simulink model "EiH_VFC_Renew_R2021b"  (R2021b)
settings: Solver=ode4  StartTime=0.0  StopTime=30  FixedStep=0.01  RelTol=1e-3
values from neighbouring files (symbols this model uses):
  denomi_threshold = 1e-8    (= 1e-08)    [param_EiH_VFC.m]
  Keo1 = Keo_Gain    (= 0.5)    [param_EiH_VFC.m]
  Keo2 = Keo_Gain    (= 0.5)    [param_EiH_VFC.m]
  Keo3 = Keo_Gain    (= 0.5)    [param_EiH_VFC.m]
  Keo4 = Keo_Gain    (= 0.5)    [param_EiH_VFC.m]
  Keo5 = Keo_Gain    (= 0.5)    [param_EiH_VFC.m]
  Keo6 = Keo_Gain    (= 0.5)    [param_EiH_VFC.m]
  pco_bar_init = pco_init + [0.15; 0.3; -0.1]    [param_EiH_VFC.m]
  pco_init = [0.0; 0.0; -1.0]    [param_EiH_VFC.m]
  Pinho_Para = [0; 0; 0; lambda_mx; lambda_my]    [param_EiH_VFC.m]
  po = [xo1; yo1; zo1; xo2; yo2; zo2; xo3; yo3; zo3; xo4; yo4; zo4]    [param_EiH_VFC.m]
  pzeta_wo_init = [pwo_init;zetawo_init]    [param_EiH_VFC.m]
  R_threshold = 1e-8    (= 1e-08)    [param_EiH_VFC.m]
  Rco_bar_init = Rfromxi(zetaco_bar_init)    [param_EiH_VFC.m]
  Rco_init = Rfromxi(zetaco_init)    [param_EiH_VFC.m]
  sx = -1.02500e5    (= -102500)    [param_EiH_VFC.m]
  sy = -1.02500e5    (= -102500)    [param_EiH_VFC.m]
  zeta_threshold = 1e-8    (= 1e-08)    [param_EiH_VFC.m]
undefined symbols (not defined in the file or in its folder): Angle, Axis, Km1, Km2, Km3, Km4, Km5, Km6, magnitude, pzeta_md
libraries: dspmtrx3 x2, robotcorelib x1, vrlib x1
(part 1 of 4)
settings Model: Creator=toshiyuki  LastModifiedBy=takeh
settings SolverCC: AlgebraicLoopSolver=TrustRegion
settings DataIOCC: ReturnWorkspaceOutputs=off
settings DebuggingCC: SFMachineParentedDataDiag=warning  ArithmeticOperatorsInVariantConditions=warning
settings SFSimCC: SimUseLocalCustomCode=off  CustomCodeUndefinedFunction=UseInterfaceOnly
settings RTWCC: RTWUseLocalCustomCode=off

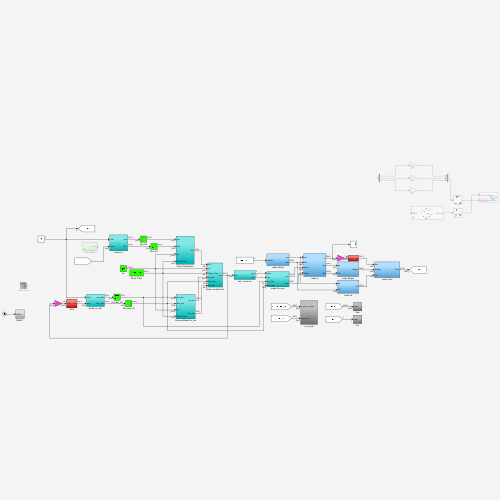
[thumbnail: Simulink's stored preview of the top-level diagram]
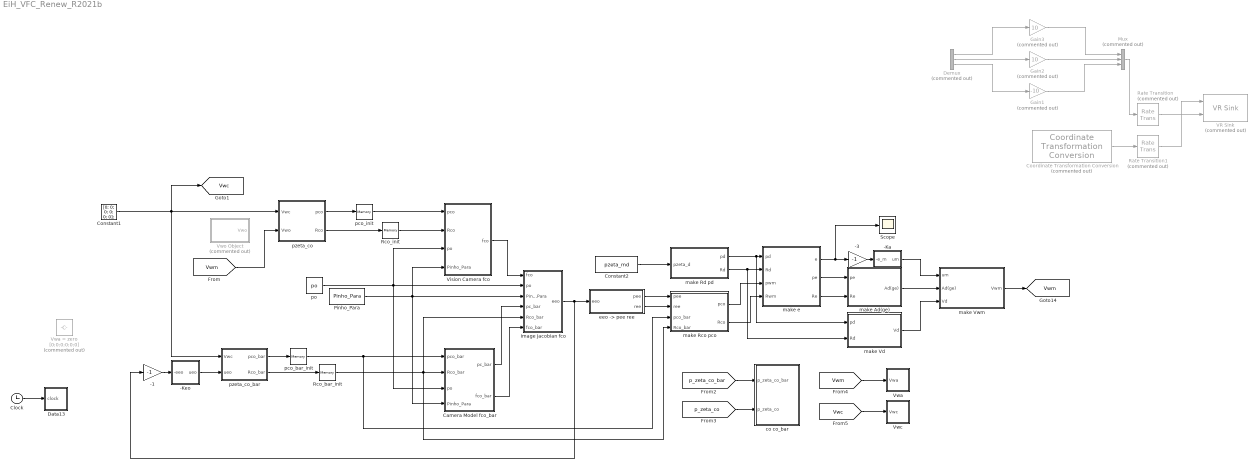
== system EiH_VFC_Renew_R2021b ==
  -1 : Gain  Gain=-1  SaturateOnIntegerOverflow=on  OutDataTypeStr=Inherit: Same as input  ParamDataTypeStr=Inherit: Same as input
  -3 : Gain  Gain=-1  SaturateOnIntegerOverflow=on  OutDataTypeStr=Inherit: Same as input  ParamDataTypeStr=Inherit: Same as input
  -Ka : Subsystem
  -Keo : Subsystem
  Camera Model fco_bar : Subsystem
  Clock : Clock
  Constant1 : Constant  Value=[0; 0; 0; 0; 0; 0];
  Constant2 : Constant  Value=pzeta_md
  Coordinate Transformation Conversion : robotcorelib/Coordinate Transformation Conversion  Commented=on  InputRepresentation=Rotation Matrix  InputEulerSequence=ZYX  ShowTrVecInputPort=on  OutputRepresentation=Axis-Angle  OutputEulerSequence=ZYX  ShowTrVecOutputPort=on  SimulateUsing=Interpreted execution
      settings: SourceProductBaseCode=NV,RO,RR,UV
  Data13 : Subsystem
  Demux : Demux  Commented=on  Outputs=3
  Gain1 : Gain  Commented=on  Gain=-10
  Gain2 : Gain  Commented=on  Gain=10
  Gain3 : Gain  Commented=on  Gain=10
  Image Jacobian fco : Subsystem
  Mux : Mux  Commented=on  Inputs=3
  "Pinho_Para " : Constant  Value=Pinho_Para  VectorParams1D=off
  Rate Transition : RateTransition  Commented=on
  Rate Transition1 : RateTransition  Commented=on
  Rco_bar_init : Memory  InitialCondition=Rco_bar_init
  Rco_init : Memory  InitialCondition=Rco_init
  Scope : Scope
  VR Sink : vrlib/VR Sink  Commented=on  InstantiateOnLoad=on  SampleTime=0.1  ViewEnable=on  RemoteChange=off  RemoteView=off  FieldsWritten=drone.rotation.4.1.1.double#drone.translation.3.1.1.double  WorldFileName=Drone.wrl  WorldDescription=drone  AutoView=off  VideoDimensions=[]  AllowVariableSize=off
  Vision Camera fco : Subsystem
  Vwa : Subsystem
  Vwa = zero : Constant  Commented=on  Value=[0;0;0;0;0;0]  VectorParams1D=off
  Vwc : Subsystem
  Vwo Object : Subsystem  Commented=on
  co co_bar : Subsystem
  "eeo -> pee ree" : Subsystem
  make Ad(ge) : Subsystem
  make Rco pco : Subsystem
  make Rd pd : Subsystem
  make Vd : Subsystem
  make Vwm : Subsystem
  make e : Subsystem
  pco_bar_init : Memory  InitialCondition=pco_bar_init
  pco_init : Memory  InitialCondition=pco_init
  "po " : Constant  Value=po  VectorParams1D=off
  pzeta_co : Subsystem
  pzeta_co_bar : Subsystem
  tag scope: Vwc=global, Vwm=global
  wires:
  Constant1/1 -> pzeta_co/1(Vwc), [Vwc], pzeta_co_bar/1(Vwc)
  pzeta_co_bar/1(" pco_bar") -> pco_bar_init/1
  Vision Camera fco/1(fco) -> Image Jacobian fco/1(fco)
  -Keo/1(ueo) -> pzeta_co_bar/2(ueo)
  -1/1 -> -Keo/1(-eeo)
  pzeta_co/1(" pco") -> pco_init/1
  Rco_init/1 -> Vision Camera fco/2(Rco)
  pco_init/1 -> Vision Camera fco/1(pco)
  pzeta_co/2(" Rco") -> Rco_init/1
  Camera Model fco_bar/2(fco_bar) -> Image Jacobian fco/6(fco_bar)
  "po "/1 -> Camera Model fco_bar/3(po), Image Jacobian fco/2(po), Vision Camera fco/3(po)
  Rco_bar_init/1 -> Camera Model fco_bar/2(Rco_bar), make Rco pco/4(Rco_bar), Image Jacobian fco/5(Rco_bar)
  "Pinho_Para "/1 -> Camera Model fco_bar/4(Pinho_Para), Vision Camera fco/4(Pinho_Para), Image Jacobian fco/3(Pinho_Para)
  pco_bar_init/1 -> make Rco pco/3(pco_bar), Camera Model fco_bar/1(pco_bar)
  pzeta_co_bar/2(" Rco_bar") -> Rco_bar_init/1
  Camera Model fco_bar/1(pc_bar) -> Image Jacobian fco/4(pc_bar)
  Clock/1 -> Data13/1(clock)
  Image Jacobian fco/1(eeo) -> "eeo -> pee ree"/1(eeo), -1/1
  make Rco pco/2(Rco) -> make e/4(Rwm)
  -3/1 -> -Ka/1(-e_m)
  make e/1(e) -> Scope/1, -3/1
  make Rco pco/1(pco) -> make e/3(pwm)
  [p_zeta_co_bar] -> co co_bar/1(p_zeta_co_bar)
  [p_zeta_co] -> co co_bar/2(p_zeta_co)
  "eeo -> pee ree"/1(pee) -> make Rco pco/1(pee)
  "eeo -> pee ree"/2(ree) -> make Rco pco/2(ree)
  [Vwm] -> Vwa/1(Vwa)
  [Vwc] -> Vwc/1(Vwc)
  Coordinate Transformation Conversion/1 -> Rate Transition1/1
  Rate Transition/1 -> VR Sink/2
  Rate Transition1/1 -> VR Sink/1
  Demux/3 -> Gain1/1
  Gain1/1 -> Mux/3
  Demux/2 -> Gain2/1
  Demux/1 -> Gain3/1
  Mux/1 -> Rate Transition/1
  Gain2/1 -> Mux/2
  Gain3/1 -> Mux/1
  Constant2/1 -> make Rd pd/1(pzeta_d)
  make Rd pd/1(pd) -> make Vd/1(pd), make e/1(pd)
  make Rd pd/2(Rd) -> make Vd/2(Rd), make e/2(Rd)
  make e/2(pe) -> make Ad(ge)/1(pe)
  make e/3(Re) -> make Ad(ge)/2(Re)
  make Ad(ge)/1(Ad(ge)) -> make Vwm/2(Ad(ge))
  -Ka/1(um) -> make Vwm/1(um)
  make Vd/1(Vd) -> make Vwm/3(Vd)
  make Vwm/1(Vwm) -> [Vwm]
  [Vwm] -> pzeta_co/2(Vwo)

== system EiH_VFC_Renew_R2021b/-Ka ==
  -e_m : Inport
  Data um : Subsystem
  Gain : Gain  Gain=-1  Multiplication=Matrix(K*u)  SaturateOnIntegerOverflow=on  OutDataTypeStr=Inherit: Same as input  ParamDataTypeStr=Inherit: Same as input
  Kcc : Subsystem
  Product : Product  Multiplication=Matrix(*)  InputSameDT=on  SaturateOnIntegerOverflow=on  OutDataTypeStr=Inherit: Same as first input
  um WS : Subsystem
  um : Outport  VectorParamsAs1DForOutWhenUnconnected=off
  wires:
  Gain/1 -> Product/1
  Kcc/1(Km) -> Gain/1
  -e_m/1 -> Product/2
  Product/1 -> um WS/1(um), Data um/1(um), um/1

== system EiH_VFC_Renew_R2021b/-Keo ==
  -eeo : Inport
  Data ueo : Subsystem
  Gain : Gain  Gain=-1  Multiplication=Matrix(K*u)  SaturateOnIntegerOverflow=on  OutDataTypeStr=Inherit: Same as input  ParamDataTypeStr=Inherit: Same as input
  Keo : Subsystem
  Product : Product  Multiplication=Matrix(*)  InputSameDT=on  SaturateOnIntegerOverflow=on  OutDataTypeStr=Inherit: Same as first input
  ueo WS : Subsystem
  ueo : Outport  VectorParamsAs1DForOutWhenUnconnected=off
  wires:
  Gain/1 -> Product/1
  Keo/1(Keo) -> Gain/1
  -eeo/1 -> Product/2
  Product/1 -> Data ueo/1(ueo), ueo WS/1(ueo), ueo/1

== system EiH_VFC_Renew_R2021b/Camera Model fco_bar ==
  pco_bar : Inport
  Rco_bar : Inport  Port=2
  po : Inport  Port=3
  Pinho_Para : Inport  Port=4
  " fcq " : Subsystem
  Data fco_bar : Subsystem
  Feature Point Model : Subsystem
  fco_bar WS : Subsystem
  make p_zeta_co_bar : Subsystem
  pc_bar : Outport  VectorParamsAs1DForOutWhenUnconnected=off
  fco_bar : Outport  Port=2  VectorParamsAs1DForOutWhenUnconnected=off
  wires:
  Feature Point Model/1(pc) -> " fcq "/1(pc), pc_bar/1
  pco_bar/1 -> Feature Point Model/1(pcq), make p_zeta_co_bar/1(pco_bar)
  Rco_bar/1 -> make p_zeta_co_bar/2(Rco_bar), Feature Point Model/2(Rcq)
  po/1 -> Feature Point Model/3(pq)
  Pinho_Para/1 -> " fcq "/2(Pinho_Para)
  " fcq "/1(fcq) -> Data fco_bar/1(fco_bar), fco_bar WS/1(fco_bar), fco_bar/1

== system EiH_VFC_Renew_R2021b/Data13 ==
  clock : Inport
  To Workspace1 : ToWorkspace  VariableName=clock  SaveFormat=Structure  SampleTime=-1
  wires:
  clock/1 -> To Workspace1/1

== system EiH_VFC_Renew_R2021b/Image Jacobian fco ==
  fco : Inport
  po : Inport  Port=2
  Pinho_Para : Inport  Port=3
  pc_bar : Inport  Port=4
  Rco_bar : Inport  Port=5
  fco_bar : Inport  Port=6
  Data eeo : Subsystem
  Image Jacobian : Subsystem
  eeo WS : Subsystem
  maka ee : Subsystem
  pseudo inverse : Subsystem
  eeo : Outport  VectorParamsAs1DForOutWhenUnconnected=off
  wires:
  pseudo inverse/1(J_daggar) -> maka ee/1(J_daggar)
  Image Jacobian/1(J) -> pseudo inverse/1(J)
  Pinho_Para/1 -> Image Jacobian/2(Pinho_Para)
  Rco_bar/1 -> Image Jacobian/3(Rcq_bar)
  fco/1 -> maka ee/2(f)
  po/1 -> Image Jacobian/4(pq)
  fco_bar/1 -> maka ee/3(f_bar)
  pc_bar/1 -> Image Jacobian/1(pc_bar)
  maka ee/1(ee) -> eeo/1, Data eeo/1(eeo), eeo WS/1(eeo)

== system EiH_VFC_Renew_R2021b/Vision Camera fco ==
  pco : Inport
  Rco : Inport  Port=2
  po : Inport  Port=3
  Pinho_Para : Inport  Port=4
  " fcq " : Subsystem
  Data fco : Subsystem
  Feature Point Model : Subsystem
  fco WS : Subsystem
  make pzeta co : Subsystem
  fco : Outport  VectorParamsAs1DForOutWhenUnconnected=off
  wires:
  Feature Point Model/1(pc) -> " fcq "/1(pc)
  pco/1 -> make pzeta co/1("pco "), Feature Point Model/1(pcq)
  Rco/1 -> make pzeta co/2(Rco), Feature Point Model/2(Rcq)
  po/1 -> Feature Point Model/3(pq)
  Pinho_Para/1 -> " fcq "/2(Pinho_Para)
  " fcq "/1(fcq) -> Data fco/1(fco), fco WS/1(fco), fco/1

== system EiH_VFC_Renew_R2021b/Vwa ==
  Vwa : Inport
  Demux : Demux  Outputs=6
      settings: DisplayOption=none
  Demux1 : Demux
      settings: DisplayOption=none
  Gain : Gain  Gain=1/0.05
  Gain1 : Gain  Gain=1/0.05
  Gain2 : Gain  Gain=1/0.01
  Gain3 : Gain  Gain=1/0.015
  Mux : Mux
  Mux1 : Mux
  V wa : Scope
  Vwa Param : Scope
  "Vwa1 " : Scope
  Vwa{2..6} (5 alike) : Scope
  wires:
  Demux/4 -> Vwa4/1
  Demux/1 -> "Vwa1 "/1, Mux/1
  Demux/2 -> Mux/2, Vwa2/1
  Vwa/1 -> Demux/1
  Demux/3 -> Mux/3, Vwa3/1
  Demux/5 -> Vwa5/1
  Demux/6 -> Mux/4, Vwa6/1
  Mux/1 -> Demux1/1, V wa/1
  Demux1/1 -> Gain/1
  Gain/1 -> Mux1/1
  Demux1/2 -> Gain1/1
  Demux1/3 -> Gain2/1
  Gain1/1 -> Mux1/2
  Gain2/1 -> Mux1/3
  Demux1/4 -> Gain3/1
  Gain3/1 -> Mux1/4
  Mux1/1 -> Vwa Param/1

== system EiH_VFC_Renew_R2021b/Vwc ==
  Vwc : Inport
  Demux : Demux  Outputs=6
      settings: DisplayOption=none
  Mux : Mux
  V wc : Scope
  "Vwc1 " : Scope
  Vwc{2..6} (5 alike) : Scope
  wires:
  Demux/4 -> Vwc4/1
  Demux/1 -> "Vwc1 "/1, Mux/1
  Demux/2 -> Mux/2, Vwc2/1
  Vwc/1 -> Demux/1
  Demux/3 -> Mux/3, Vwc3/1
  Demux/5 -> Vwc5/1
  Demux/6 -> Mux/4, Vwc6/1
  Mux/1 -> V wc/1

== system EiH_VFC_Renew_R2021b/Vwo Object ==
  Data Vwo : Subsystem
  Data pwo : Subsystem
  Data zetawo : Subsystem
  Demux : Demux  Outputs=2
      settings: DisplayOption=none
  Demux1 : Demux  Outputs=2
      settings: DisplayOption=none
  Math Function : Math  Operator=transpose  SignedPower=on  SaturateOnIntegerOverflow=on
  Mux : Mux  Inputs=2
  Product : Product  Multiplication=Matrix(*)  SaturateOnIntegerOverflow=on  OutDataTypeStr=Inherit: Same as first input
  Product1 : Product  Multiplication=Matrix(*)  SaturateOnIntegerOverflow=on  OutDataTypeStr=Inherit: Same as first input
  RfromW : MATLABFcn  MATLABFcn=RfromW  OutputDimensions=[3,3]  OutputSignalType=real  Output1D=off
  Vwo WS : Subsystem
  Vwo1 : Derivative
  Vwo3 : Derivative
  highspeed_exp_object_motion : Subsystem
  pwo WS : Subsystem
  vee : Subsystem
  zetawo WS : Subsystem
  Vwo : Outport  VectorParamsAs1DForOutWhenUnconnected=off
  wires:
  highspeed_exp_object_motion/1(pwo & xiwo) -> Demux1/1, Demux/1
  Demux/2 -> RfromW/1
  RfromW/1 -> Vwo1/1, Math Function/1
  Demux/1 -> Vwo3/1
  Math Function/1 -> Product/1, Product1/1
  Vwo3/1 -> Product/2
  Vwo1/1 -> Product1/2
  Product1/1 -> vee/1("[3*3]")
  Product/1 -> Mux/1
  vee/1("[3*1]") -> Mux/2
  Mux/1 -> Vwo WS/1(Vwo), Data Vwo/1(Vwo), Vwo/1
  Demux1/1 -> Data pwo/1(pwo), pwo WS/1(pwo)
  Demux1/2 -> Data zetawo/1(zeta wo), zetawo WS/1(zetawo)

== system EiH_VFC_Renew_R2021b/co co_bar ==
  p_zeta_co_bar : Inport
  p_zeta_co : Inport  Port=2
  Demux : Demux  Outputs=6
  Demux1 : Demux  Outputs=6
  Sum : Sum  Inputs=+-
  px : Scope  NumInputPorts=2
  py : Scope  NumInputPorts=2
  pz : Scope  NumInputPorts=2
  pzetaco pzetaco_bar : Scope  NumInputPorts=2
  "pzetaco pzetaco_bar error " : Scope
  zetax : Scope  NumInputPorts=2
  zetay : Scope  NumInputPorts=2
  zetaz : Scope  NumInputPorts=2
  wires:
  p_zeta_co_bar/1 -> pzetaco pzetaco_bar/1, Sum/1, Demux/1
  p_zeta_co/1 -> pzetaco pzetaco_bar/2, Sum/2, Demux1/1
  Demux/1 -> px/1
  Demux1/1 -> px/2
  Demux/2 -> py/1
  Demux1/2 -> py/2
  Demux/3 -> pz/1
  Demux1/3 -> pz/2
  Demux/4 -> zetax/1
  Demux1/4 -> zetax/2
  Demux/5 -> zetay/1
  Demux1/5 -> zetay/2
  Demux/6 -> zetaz/1
  Demux1/6 -> zetaz/2
  Sum/1 -> "pzetaco pzetaco_bar error "/1

== system EiH_VFC_Renew_R2021b/eeo -> pee ree ==
  eeo : Inport
  Demux : Demux  Outputs=6
  Mux : Mux  Inputs=3
  Mux1 : Mux  Inputs=3
  pee : Outport  VectorParamsAs1DForOutWhenUnconnected=off
  ree : Outport  Port=2  VectorParamsAs1DForOutWhenUnconnected=off
  wires:
  eeo/1 -> Demux/1
  Demux/1 -> Mux/1
  Demux/2 -> Mux/2
  Demux/3 -> Mux/3
  Mux/1 -> pee/1
  Mux1/1 -> ree/1
  Demux/4 -> Mux1/1
  Demux/5 -> Mux1/2
  Demux/6 -> Mux1/3

== system EiH_VFC_Renew_R2021b/make Ad(ge) ==
  note: $\hat{p_e}R_e$
  note: $\left(R_e\ \hat{p_e}R_e\right)$
  note: $\left(0\ R_e\right)$
  note: $\text{Ad}_{(g_e)}=\left[\begin{array}{cc} R_e & \hat{p_e}R_e\\ 0&R_e \end{array}\right]$
  pe : Inport
  Re : Inport  Port=2
  Gain : Gain  Gain=0  Multiplication=Matrix(K*u)
  Identity Matrix : dspmtrx3/Identity Matrix  Inherit=off  N=3  Ts=1  dataType=double  isSigned=on  wordLen=16  udDataType=sfix(16)  fracBitsMode=Best precision  numFracBits=15  OutDataTypeStr=double  LastOutDataTypeStr=double
  Matrix Concatenate : Concatenate  Mode=Multidimensional array  ConcatenateDimension=2
  Matrix Concatenate1 : Concatenate  Mode=Multidimensional array  ConcatenateDimension=2
  Matrix Concatenate2 : Concatenate  Mode=Multidimensional array
  Product2 : Product  Multiplication=Matrix(*)
  wedge : Subsystem
  Ad(ge) : Outport  VectorParamsAs1DForOutWhenUnconnected=off
  wires:
  pe/1 -> wedge/1("[3x1]")
  wedge/1("[3x3]") -> Product2/1
  Re/1 -> Matrix Concatenate1/2, Product2/2, Matrix Concatenate/1
  Product2/1 -> Matrix Concatenate/2
  Matrix Concatenate/1 -> Matrix Concatenate2/1
  Matrix Concatenate1/1 -> Matrix Concatenate2/2
  Matrix Concatenate2/1 -> Ad(ge)/1
  Identity Matrix/1 -> Gain/1
  Gain/1 -> Matrix Concatenate1/1

== system EiH_VFC_Renew_R2021b/make Rco pco ==
  pee : Inport
  ree : Inport  Port=2
  pco_bar : Inport  Port=3
  Rco_bar : Inport  Port=4
  I_3 : dspmtrx3/Identity Matrix  Inherit=off  N=3  Ts=1  dataType=double  isSigned=on  wordLen=16  udDataType=sfix(16)  fracBitsMode=Best precision  numFracBits=15  OutDataTypeStr=double  LastOutDataTypeStr=double
  Product : Product  Multiplication=Matrix(*)
  Product1 : Product  Multiplication=Matrix(*)
  Sum : Sum  Inputs=|++
  Sum1 : Sum  Inputs=|++
  make p_zeta co : Subsystem
  wedge : Subsystem
  pco : Outport  VectorParamsAs1DForOutWhenUnconnected=off
  Rco : Outport  Port=2  VectorParamsAs1DForOutWhenUnconnected=off
  wires:
  wedge/1("[3x3]") -> Sum/1
  I_3/1 -> Sum/2
  Sum/1 -> Product/2
  Product/1 -> make p_zeta co/2(Rco), Rco/1
  Sum1/1 -> make p_zeta co/1("pco "), pco/1
  Product1/1 -> Sum1/2
  pco_bar/1 -> Sum1/1
  pee/1 -> Product1/2
  Rco_bar/1 -> Product1/1, Product/1
  ree/1 -> wedge/1("[3x1]")

== system EiH_VFC_Renew_R2021b/make Rd pd ==
  note: 目標姿勢
  note: 目標位置
  note: $p_d=\left(p_x \ p_y\ p_z\right)^T$$
  note: $\zeta_d=\left(\zeta_x \ \zeta_y\ \zeta_z\right)^T\text{\ \ →\ \ 回転行列}R_d$
  pzeta_d : Inport
  Demux3 : Demux  Outputs=6
      settings: DisplayOption=none
  Mux : Mux  Inputs=3
  Mux1 : Mux  Inputs=3
  make_Rd : Subsystem
  pd : Outport  VectorParamsAs1DForOutWhenUnconnected=off
  Rd : Outport  Port=2  VectorParamsAs1DForOutWhenUnconnected=off
  wires:
  Demux3/2 -> Mux1/2
  Demux3/1 -> Mux1/1
  Demux3/5 -> Mux/2
  Demux3/4 -> Mux/1
  pzeta_d/1 -> Demux3/1
  Mux/1 -> make_Rd/1(zeta_d)
  Demux3/3 -> Mux1/3
  Demux3/6 -> Mux/3
  Mux1/1 -> pd/1
  make_Rd/1(Rd) -> Rd/1

== system EiH_VFC_Renew_R2021b/make Vd ==
  note: $v_d^b=R_{d}^T\dot{p}_{d}$
  note: $\omega_d^b=\left(R_{d}^T\dot{R}_{d}\right)^\vee$
  note: $V_d^b=\left[\begin{array}{c} v_d^b\\ \omega_d^b \end{array} \right]$
  pd : Inport
  Rd : Inport  Port=2
  Derivative : Derivative
  Derivative1 : Derivative
  Math Function : Math  Operator=transpose  SignedPower=on  SaturateOnIntegerOverflow=on
  Mux : Mux  Inputs=2
  Product1 : Product  Multiplication=Matrix(*)
  Product2 : Product  Multiplication=Matrix(*)
  vee : Subsystem
  Vd : Outport  VectorParamsAs1DForOutWhenUnconnected=off
  wires:
  pd/1 -> Derivative/1
  Rd/1 -> Derivative1/1, Math Function/1
  Math Function/1 -> Product2/1, Product1/1
  Derivative1/1 -> Product1/2
  Product1/1 -> vee/1("[3*3]")
  vee/1("[3*1]") -> Mux/2
  Product2/1 -> Mux/1
  Mux/1 -> Vd/1
  Derivative/1 -> Product2/2

== system EiH_VFC_Renew_R2021b/make Vwm ==
  note: $\text{Ad}_{(g_e)}\ \ \text{→}\ \ \text{Ad}_{(g_e)}^{-1}$
  note: $V_{wm}=-\text{Ad}_{(g_e)}^{-1}\left(u_m-V_d\right)$
  um : Inport
  Ad(ge) : Inport  Port=2
  Vd : Inport  Port=3
  -3 : Gain  Gain=-1  SaturateOnIntegerOverflow=on  OutDataTypeStr=Inherit: Same as input  ParamDataTypeStr=Inherit: Same as input
  MATLAB Function : MATLAB Function  TreatAsAtomicUnit=on
  Product2 : Product  Multiplication=Matrix(*)
  Sum : Sum  Inputs=|+-
  Vwm : Outport  VectorParamsAs1DForOutWhenUnconnected=off
  wires:
  Product2/1 -> Vwm/1
  Ad(ge)/1 -> MATLAB Function/1(Ad_ge)
  um/1 -> Sum/1
  Vd/1 -> Sum/2
  MATLAB Function/1(inv_Ad_ge) -> -3/1
  -3/1 -> Product2/1
  Sum/1 -> Product2/2

== system EiH_VFC_Renew_R2021b/make e ==
  note: 制御偏差ベクトル
  note: 姿勢偏差ベクトル
  note: 姿勢偏差
  note: 位置偏差ベクトル
  note: $p_e=R_d^T\left (p_{wm}-p_d\right)$
  note: $R_e=R_d^TR_{wm}$
  note: $r_e=\frac{1}{2}\left(R_e-R_e^T\right)^\vee$
  note: $e=\left(p_e\ r_e)^T$
  pd : Inport
  Rd : Inport  Port=2
  pwm : Inport  Port=3
  Rwm : Inport  Port=4
  Gain : Gain  Gain=1/2
  Math Function : Math  Operator=transpose  SignedPower=on  SaturateOnIntegerOverflow=on
  Math Function1 : Math  Operator=transpose  SignedPower=on  SaturateOnIntegerOverflow=on
  Mux : Mux  Inputs=2
  Product1 : Product  Multiplication=Matrix(*)
  Product2 : Product  Multiplication=Matrix(*)
  Sum : Sum  Inputs=|+-
  Sum1 : Sum  Inputs=|+-
  vee : Subsystem
  e : Outport  VectorParamsAs1DForOutWhenUnconnected=off
  pe : Outport  Port=2  VectorParamsAs1DForOutWhenUnconnected=off
  Re : Outport  Port=3  VectorParamsAs1DForOutWhenUnconnected=off
  wires:
  Rd/1 -> Math Function/1
  Math Function/1 -> Product2/1, Product1/1
  Rwm/1 -> Product1/2
  pwm/1 -> Sum1/1
  pd/1 -> Sum1/2
  Sum1/1 -> Product2/2
  vee/1("[3*1]") -> Mux/2
  Sum/1 -> Gain/1
  Math Function1/1 -> Sum/2
  Product2/1 -> pe/1, Mux/1
  Gain/1 -> vee/1("[3*3]")
  Mux/1 -> e/1
  Product1/1 -> Re/1, Math Function1/1, Sum/1

== system EiH_VFC_Renew_R2021b/pzeta_co ==
  Vwc : Inport
  Vwo : Inport  Port=2
  "  wedge  " : Subsystem
  " wedge " : Subsystem
  Demux1 : Demux  Outputs=2
      settings: DisplayOption=none
  Demux2 : Demux  Outputs=2
      settings: DisplayOption=none
  Product{1..4} (4 alike) : Product  Multiplication=Matrix(*)  InputSameDT=on  SaturateOnIntegerOverflow=on  OutDataTypeStr=Inherit: Same as first input
  Sum1 : Sum  Inputs=|-+  InputSameDT=on  SaturateOnIntegerOverflow=on  OutDataTypeStr=Inherit: Same as first input
  Sum9 : Sum  Inputs=-++  InputSameDT=on  SaturateOnIntegerOverflow=on  OutDataTypeStr=Inherit: Same as first input
  dot Rco : Integrator  InitialCondition=Rco_init
  dot pco : Integrator  InitialCondition=pco_init
  wedge : Subsystem
  " pco" : Outport  VectorParamsAs1DForOutWhenUnconnected=off
  " Rco" : Outport  Port=2  VectorParamsAs1DForOutWhenUnconnected=off
  wires:
  Sum1/1 -> dot Rco/1
  Product4/1 -> Sum1/2
  Product3/1 -> Sum1/1
  "  wedge  "/1("[3x3]") -> Product4/2
  Demux2/2 -> "  wedge  "/1("[3x1]")
  " wedge "/1("[3x3]") -> Product3/1
  Demux2/1 -> Product2/2
  Demux1/2 -> " wedge "/1("[3x1]"), Product1/2
  wedge/1("[3x3]") -> Product1/1
  Product2/1 -> Sum9/3
  Product1/1 -> Sum9/2
  Sum9/1 -> dot pco/1
  Demux1/1 -> Sum9/1
  Vwo/1 -> Demux2/1
  dot Rco/1 -> Product2/1, Product3/2, Product4/1, " Rco"/1
  Vwc/1 -> Demux1/1
  dot pco/1 -> wedge/1("[3x1]"), " pco"/1

== system EiH_VFC_Renew_R2021b/pzeta_co_bar ==
  Vwc : Inport
  ueo : Inport  Port=2
  "  wedge  " : Subsystem
  " wedge " : Subsystem
  Demux1 : Demux  Outputs=2
      settings: DisplayOption=none
  Demux2 : Demux  Outputs=2
      settings: DisplayOption=none
  Product{1..4} (4 alike) : Product  Multiplication=Matrix(*)  InputSameDT=on  SaturateOnIntegerOverflow=on  OutDataTypeStr=Inherit: Same as first input
  Sum1 : Sum  Inputs=|-+  InputSameDT=on  SaturateOnIntegerOverflow=on  OutDataTypeStr=Inherit: Same as first input
  Sum9 : Sum  Inputs=-++  InputSameDT=on  SaturateOnIntegerOverflow=on  OutDataTypeStr=Inherit: Same as first input
  dot Rco_bar : Integrator  InitialCondition=Rco_bar_init
  dot pco_bar : Integrator  InitialCondition=pco_bar_init
  wedge : Subsystem
  " pco_bar" : Outport  VectorParamsAs1DForOutWhenUnconnected=off
  " Rco_bar" : Outport  Port=2  VectorParamsAs1DForOutWhenUnconnected=off
  wires:
  dot pco_bar/1 -> " pco_bar"/1, wedge/1("[3x1]")
  Vwc/1 -> Demux1/1
  dot Rco_bar/1 -> " Rco_bar"/1, Product4/1, Product3/2, Product2/1
  ueo/1 -> Demux2/1
  Demux1/1 -> Sum9/1
  Sum9/1 -> dot pco_bar/1
  Product1/1 -> Sum9/2
  Product2/1 -> Sum9/3
  wedge/1("[3x3]") -> Product1/1
  Demux1/2 -> Product1/2, " wedge "/1("[3x1]")
  Demux2/1 -> Product2/2
  " wedge "/1("[3x3]") -> Product3/1
  Demux2/2 -> "  wedge  "/1("[3x1]")
  "  wedge  "/1("[3x3]") -> Product4/2
  Product3/1 -> Sum1/1
  Product4/1 -> Sum1/2
  Sum1/1 -> dot Rco_bar/1

== system EiH_VFC_Renew_R2021b/-Ka/Data um ==
  um : Inport
  Demux : Demux  Outputs=6
      settings: DisplayOption=none
  "ua1 " : Scope
  ua{2..6} (5 alike) : Scope
  wires:
  Demux/4 -> ua4/1
  Demux/1 -> "ua1 "/1
  Demux/2 -> ua2/1
  um/1 -> Demux/1
  Demux/3 -> ua3/1
  Demux/5 -> ua5/1
  Demux/6 -> ua6/1

== system EiH_VFC_Renew_R2021b/-Ka/Kcc ==
  Ke1 : Constant  Value=Km1
  Ke2 : Constant  Value=Km2
  Ke3 : Constant  Value=Km3
  Ke4 : Constant  Value=Km4
  Ke5 : Constant  Value=Km5
  Ke6 : Constant  Value=Km6
  Mux : Mux  Inputs=6
  diag : Subsystem
  Km : Outport  VectorParamsAs1DForOutWhenUnconnected=off
  wires:
  Mux/1 -> diag/1(in[6*1])
  Ke6/1 -> Mux/6
  Ke5/1 -> Mux/5
  Ke4/1 -> Mux/4
  Ke3/1 -> Mux/3
  Ke2/1 -> Mux/2
  Ke1/1 -> Mux/1
  diag/1(diag) -> Km/1

== system EiH_VFC_Renew_R2021b/-Ka/um WS ==
  um : Inport
  Clock : Clock
  Demux4 : Demux  Outputs=6
      settings: DisplayOption=none
  Mux2 : Mux  Inputs=7
  To Workspace1 : ToWorkspace  VariableName=um  SaveFormat=Structure  SampleTime=-1
  wires:
  Demux4/6 -> Mux2/7
  Demux4/5 -> Mux2/6
  Demux4/4 -> Mux2/5
  Demux4/3 -> Mux2/4
  Demux4/2 -> Mux2/3
  Demux4/1 -> Mux2/2
  Clock/1 -> Mux2/1
  Mux2/1 -> To Workspace1/1
  um/1 -> Demux4/1

== system EiH_VFC_Renew_R2021b/-Keo/Data ueo ==
  ueo : Inport
  Demux : Demux  Outputs=6
      settings: DisplayOption=none
  ueo{1..6} (6 alike) : Scope
  wires:
  Demux/4 -> ueo4/1
  Demux/1 -> ueo1/1
  Demux/2 -> ueo2/1
  ueo/1 -> Demux/1
  Demux/3 -> ueo3/1
  Demux/5 -> ueo5/1
  Demux/6 -> ueo6/1

== system EiH_VFC_Renew_R2021b/-Keo/Keo ==
  Ke1 : Constant  Value=Keo1
  Ke2 : Constant  Value=Keo2
  Ke3 : Constant  Value=Keo3
  Ke4 : Constant  Value=Keo4
  Ke5 : Constant  Value=Keo5
  Ke6 : Constant  Value=Keo6
  Mux : Mux  Inputs=6
  diag : Subsystem
  Keo : Outport  VectorParamsAs1DForOutWhenUnconnected=off
  wires:
  Mux/1 -> diag/1(in[6*1])
  Ke6/1 -> Mux/6
  Ke5/1 -> Mux/5
  Ke4/1 -> Mux/4
  Ke3/1 -> Mux/3
  Ke2/1 -> Mux/2
  Ke1/1 -> Mux/1
  diag/1(diag) -> Keo/1

== system EiH_VFC_Renew_R2021b/-Keo/ueo WS ==
  ueo : Inport
  Clock : Clock
  Demux4 : Demux  Outputs=6
      settings: DisplayOption=none
  Mux2 : Mux  Inputs=7
  To Workspace1 : ToWorkspace  VariableName=ueo  SaveFormat=Structure  SampleTime=-1
  wires:
  Demux4/6 -> Mux2/7
  Demux4/5 -> Mux2/6
  Demux4/4 -> Mux2/5
  Demux4/3 -> Mux2/4
  Demux4/2 -> Mux2/3
  Demux4/1 -> Mux2/2
  Clock/1 -> Mux2/1
  Mux2/1 -> To Workspace1/1
  ueo/1 -> Demux4/1

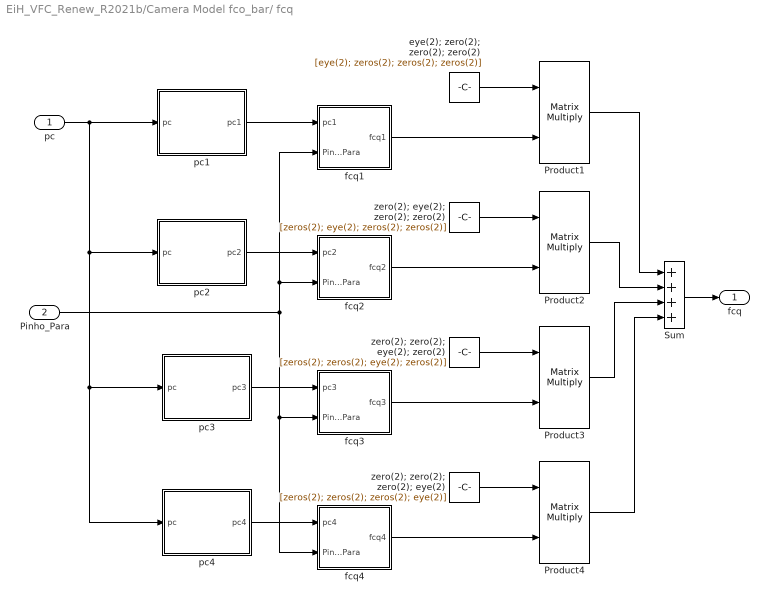
== system EiH_VFC_Renew_R2021b/Camera Model fco_bar/ fcq  ==
  pc : Inport
  Pinho_Para : Inport  Port=2
  Product{1..4} (4 alike) : Product  Multiplication=Matrix(*)  InputSameDT=on  SaturateOnIntegerOverflow=on  OutDataTypeStr=Inherit: Same as first input
  Sum : Sum  Inputs=++++  InputSameDT=on  SaturateOnIntegerOverflow=on  OutDataTypeStr=Inherit: Same as first input
  eye(2); zero(2); zero(2); zero(2) : Constant  Value=[eye(2); zeros(2); zeros(2); zeros(2)]  VectorParams1D=off
  fcq1 : Subsystem
  fcq2 : Subsystem
  fcq3 : Subsystem
  fcq4 : Subsystem
  pc1 : Subsystem
  pc2 : Subsystem
  pc3 : Subsystem
  pc4 : Subsystem
  zero(2); eye(2); zero(2); zero(2) : Constant  Value=[zeros(2); eye(2); zeros(2); zeros(2)]  VectorParams1D=off
  zero(2); zero(2); eye(2); zero(2) : Constant  Value=[zeros(2); zeros(2); eye(2); zeros(2)]  VectorParams1D=off
  zero(2); zero(2); zero(2); eye(2) : Constant  Value=[zeros(2); zeros(2); zeros(2); eye(2)]  VectorParams1D=off
  fcq : Outport  VectorParamsAs1DForOutWhenUnconnected=off
  wires:
  Pinho_Para/1 -> fcq4/2(Pinho_Para), fcq3/2(Pinho_Para), fcq2/2(Pinho_Para), fcq1/2(Pinho_Para)
  pc4/1(pc4) -> fcq4/1(pc4)
  pc3/1(pc3) -> fcq3/1(pc3)
  pc2/1(pc2) -> fcq2/1(pc2)
  Sum/1 -> fcq/1
  fcq4/1(fcq4) -> Product4/2
  fcq3/1(fcq3) -> Product3/2
  fcq2/1(fcq2) -> Product2/2
  fcq1/1(fcq1) -> Product1/2
  Product4/1 -> Sum/4
  Product2/1 -> Sum/2
  Product3/1 -> Sum/3
  Product1/1 -> Sum/1
  zero(2); zero(2); zero(2); eye(2)/1 -> Product4/1
  zero(2); zero(2); eye(2); zero(2)/1 -> Product3/1
  zero(2); eye(2); zero(2); zero(2)/1 -> Product2/1
  eye(2); zero(2); zero(2); zero(2)/1 -> Product1/1
  pc/1 -> pc4/1(pc), pc3/1(pc), pc2/1(pc), pc1/1(pc)
  pc1/1(pc1) -> fcq1/1(pc1)

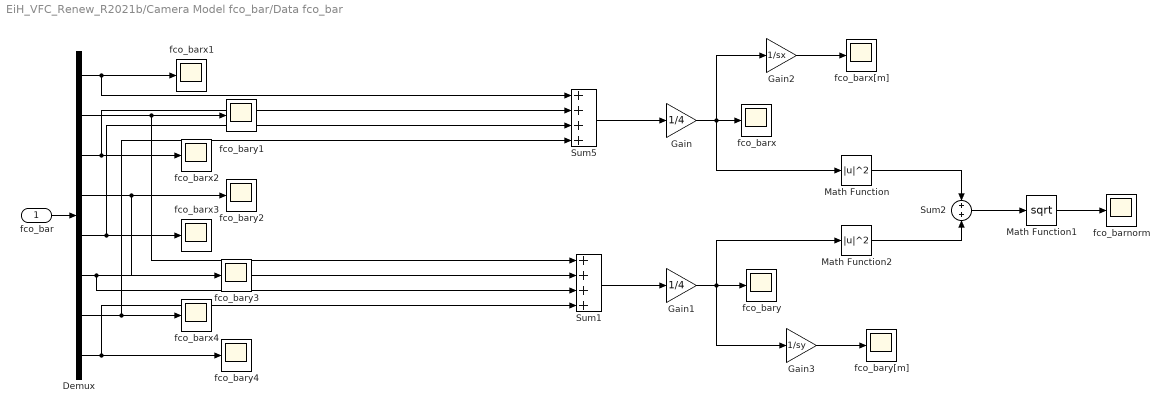
== system EiH_VFC_Renew_R2021b/Camera Model fco_bar/Data fco_bar ==
  fco_bar : Inport
  Demux : Demux  Outputs=8
      settings: DisplayOption=none
  Gain : Gain  Gain=1/4  SaturateOnIntegerOverflow=on  OutDataTypeStr=Inherit: Same as input  ParamDataTypeStr=Inherit: Same as input
  Gain1 : Gain  Gain=1/4  SaturateOnIntegerOverflow=on  OutDataTypeStr=Inherit: Same as input  ParamDataTypeStr=Inherit: Same as input
  Gain2 : Gain  Gain=1/sx  SaturateOnIntegerOverflow=on  OutDataTypeStr=Inherit: Same as input  ParamDataTypeStr=Inherit: Same as input
  Gain3 : Gain  Gain=1/sy  SaturateOnIntegerOverflow=on  OutDataTypeStr=Inherit: Same as input  ParamDataTypeStr=Inherit: Same as input
  Math Function : Math  Operator=magnitude^2  SignedPower=on  SaturateOnIntegerOverflow=on
  Math Function1 : Math  Operator=sqrt  SignedPower=on  SaturateOnIntegerOverflow=on
  Math Function2 : Math  Operator=magnitude^2  SignedPower=on  SaturateOnIntegerOverflow=on
  Sum1 : Sum  Inputs=++++  SaturateOnIntegerOverflow=on
  Sum2 : Sum  Inputs=+|+  SaturateOnIntegerOverflow=on
  Sum5 : Sum  Inputs=++++  SaturateOnIntegerOverflow=on
  fco_barnorm : Scope
  fco_barx{,1..4} (5 alike) : Scope
  fco_barx[m] : Scope
  fco_bary{,1..4} (5 alike) : Scope
  fco_bary[m] : Scope
  wires:
  Demux/8 -> fco_bary4/1, Sum1/4
  Demux/7 -> fco_barx4/1, Sum5/4
  Demux/6 -> fco_bary3/1, Sum1/3
  Demux/5 -> fco_barx3/1, Sum5/3
  Demux/3 -> Sum5/2, fco_barx2/1
  fco_bar/1 -> Demux/1
  Demux/2 -> fco_bary1/1, Sum1/1
  Demux/1 -> fco_barx1/1, Sum5/1
  Demux/4 -> fco_bary2/1, Sum1/2
  Sum5/1 -> Gain/1
  Gain/1 -> fco_barx/1, Math Function/1, Gain2/1
  Sum1/1 -> Gain1/1
  Gain1/1 -> fco_bary/1, Math Function2/1, Gain3/1
  Math Function/1 -> Sum2/1
  Math Function2/1 -> Sum2/2
  Sum2/1 -> Math Function1/1
  Math Function1/1 -> fco_barnorm/1
  Gain2/1 -> fco_barx[m]/1
  Gain3/1 -> fco_bary[m]/1

== system EiH_VFC_Renew_R2021b/Camera Model fco_bar/Feature Point Model ==
  pcq : Inport
  Rcq : Inport  Port=2
  pq : Inport  Port=3
  Product{1..4} (4 alike) : Product  Multiplication=Matrix(*)  InputSameDT=on  SaturateOnIntegerOverflow=on  OutDataTypeStr=Inherit: Same as first input
  Sum : Sum  Inputs=++++  InputSameDT=on  SaturateOnIntegerOverflow=on  OutDataTypeStr=Inherit: Same as first input
  eye(3); zero(3); zero(3); zero(3) : Constant  Value=[eye(3); zeros(3); zeros(3); zeros(3)]  VectorParams1D=off
  pc1 : Subsystem
  pc2 : Subsystem
  pc3 : Subsystem
  pc4 : Subsystem
  zero(3); eye(3); zero(3); zero(3) : Constant  Value=[zeros(3); eye(3); zeros(3); zeros(3)]  VectorParams1D=off
  zero(3); zero(3); eye(3); zero(3) : Constant  Value=[zeros(3); zeros(3); eye(3); zeros(3)]  VectorParams1D=off
  zero(3); zero(3); zero(3); eye(3) : Constant  Value=[zeros(3); zeros(3); zeros(3); eye(3)]  VectorParams1D=off
  pc : Outport  VectorParamsAs1DForOutWhenUnconnected=off
  wires:
  Product4/1 -> Sum/4
  Product2/1 -> Sum/2
  Product3/1 -> Sum/3
  Product1/1 -> Sum/1
  Sum/1 -> pc/1
  pc4/1(pc4) -> Product4/2
  zero(3); zero(3); zero(3); eye(3)/1 -> Product4/1
  pc3/1(pc3) -> Product3/2
  zero(3); zero(3); eye(3); zero(3)/1 -> Product3/1
  pc2/1(pc2) -> Product2/2
  zero(3); eye(3); zero(3); zero(3)/1 -> Product2/1
  pc1/1(pc1) -> Product1/2
  eye(3); zero(3); zero(3); zero(3)/1 -> Product1/1
  pq/1 -> pc4/3(pq), pc3/3(pq), pc2/3(pq), pc1/3(pq)
  pcq/1 -> pc4/1(pcq), pc3/1(pcq), pc2/1(pcq), pc1/1(pcq)
  Rcq/1 -> pc4/2(Rcq), pc3/2(Rcq), pc2/2(Rcq), pc1/2(Rcq)

== system EiH_VFC_Renew_R2021b/Camera Model fco_bar/fco_bar WS ==
  fco_bar : Inport
  Clock : Clock
  Demux4 : Demux  Outputs=8
      settings: DisplayOption=none
  Mux2 : Mux  Inputs=9
  To Workspace1 : ToWorkspace  VariableName=fco_bar  SaveFormat=Structure  SampleTime=-1
  wires:
  Demux4/8 -> Mux2/9
  Demux4/7 -> Mux2/8
  Demux4/6 -> Mux2/7
  Demux4/5 -> Mux2/6
  Demux4/4 -> Mux2/5
  Demux4/3 -> Mux2/4
  Demux4/2 -> Mux2/3
  Demux4/1 -> Mux2/2
  Clock/1 -> Mux2/1
  Mux2/1 -> To Workspace1/1
  fco_bar/1 -> Demux4/1

== system EiH_VFC_Renew_R2021b/Camera Model fco_bar/make p_zeta_co_bar ==
  pco_bar : Inport
  Rco_bar : Inport  Port=2
  Data pco_bar : Subsystem
  Data zetaco_bar : Subsystem
  Mux1 : Mux  Inputs=2
  "Rco_bar -> zeta_co_bar" : Subsystem
  Rco_bar WS : Subsystem
  pco_bar WS : Subsystem
  zetaco_bar WS : Subsystem
  tag scope: p_zeta_co_bar=global
  wires:
  pco_bar/1 -> pco_bar WS/1(pco_bar), Data pco_bar/1(pco_bar), Mux1/1
  "Rco_bar -> zeta_co_bar"/1(zeta_co_bar) -> zetaco_bar WS/1(zetaco_bar), Data zetaco_bar/1(zetaco_bar), Mux1/2
  Mux1/1 -> [p_zeta_co_bar]
  Rco_bar/1 -> Rco_bar WS/1(Rco_bar), "Rco_bar -> zeta_co_bar"/1(Rco_bar)

== system EiH_VFC_Renew_R2021b/Image Jacobian fco/Data eeo ==
  eeo : Inport
  Demux : Demux  Outputs=6
      settings: DisplayOption=none
  eeo{1..6} (6 alike) : Scope
  wires:
  Demux/4 -> eeo4/1
  Demux/1 -> eeo1/1
  Demux/2 -> eeo2/1
  eeo/1 -> Demux/1
  Demux/3 -> eeo3/1
  Demux/5 -> eeo5/1
  Demux/6 -> eeo6/1

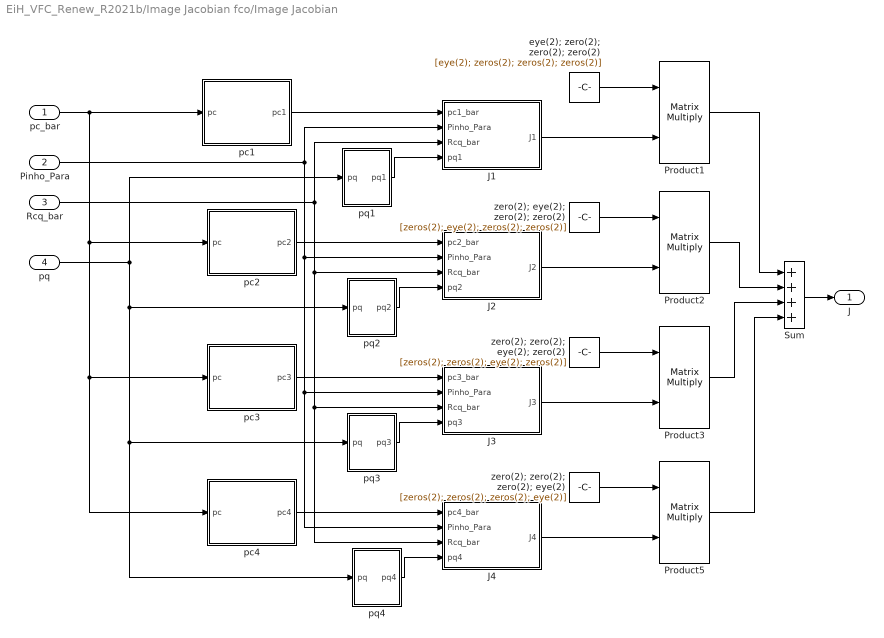
== system EiH_VFC_Renew_R2021b/Image Jacobian fco/Image Jacobian ==
  pc_bar : Inport
  Pinho_Para : Inport  Port=2
  Rcq_bar : Inport  Port=3
  pq : Inport  Port=4
  J1 : Subsystem
  J2 : Subsystem
  J3 : Subsystem
  J4 : Subsystem
  Product{1..3,5} (4 alike) : Product  Multiplication=Matrix(*)  InputSameDT=on  SaturateOnIntegerOverflow=on  OutDataTypeStr=Inherit: Same as first input
  Sum : Sum  Inputs=++++  InputSameDT=on  SaturateOnIntegerOverflow=on  OutDataTypeStr=Inherit: Same as first input
  eye(2); zero(2); zero(2); zero(2) : Constant  Value=[eye(2); zeros(2); zeros(2); zeros(2)]  VectorParams1D=off
  pc1 : Subsystem
  pc2 : Subsystem
  pc3 : Subsystem
  pc4 : Subsystem
  pq1 : Subsystem
  pq2 : Subsystem
  pq3 : Subsystem
  pq4 : Subsystem
  zero(2); eye(2); zero(2); zero(2) : Constant  Value=[zeros(2); eye(2); zeros(2); zeros(2)]  VectorParams1D=off
  zero(2); zero(2); eye(2); zero(2) : Constant  Value=[zeros(2); zeros(2); eye(2); zeros(2)]  VectorParams1D=off
  zero(2); zero(2); zero(2); eye(2) : Constant  Value=[zeros(2); zeros(2); zeros(2); eye(2)]  VectorParams1D=off
  J : Outport  VectorParamsAs1DForOutWhenUnconnected=off
  wires:
  pq/1 -> pq4/1(pq), pq3/1(pq), pq2/1(pq), pq1/1(pq)
  Rcq_bar/1 -> J1/3(Rcq_bar), J2/3(Rcq_bar), J3/3(Rcq_bar), J4/3(Rcq_bar)
  Pinho_Para/1 -> J1/2(Pinho_Para), J2/2(Pinho_Para), J4/2(Pinho_Para), J3/2(Pinho_Para)
  pc_bar/1 -> pc4/1(pc), pc3/1(pc), pc2/1(pc), pc1/1(pc)
  pc4/1(pc4) -> J4/1(pc4_bar)
  pc3/1(pc3) -> J3/1(pc3_bar)
  pq3/1(pq3) -> J3/4(pq3)
  pq4/1(pq4) -> J4/4(pq4)
  pq2/1(pq2) -> J2/4(pq2)
  pc2/1(pc2) -> J2/1(pc2_bar)
  pq1/1(pq1) -> J1/4(pq1)
  pc1/1(pc1) -> J1/1(pc1_bar)
  J4/1(J4) -> Product5/2
  Sum/1 -> J/1
  J3/1(J3) -> Product3/2
  J2/1(J2) -> Product2/2
  J1/1(J1) -> Product1/2
  Product5/1 -> Sum/4
  Product2/1 -> Sum/2
  Product3/1 -> Sum/3
  Product1/1 -> Sum/1
  zero(2); zero(2); zero(2); eye(2)/1 -> Product5/1
  zero(2); zero(2); eye(2); zero(2)/1 -> Product3/1
  zero(2); eye(2); zero(2); zero(2)/1 -> Product2/1
  eye(2); zero(2); zero(2); zero(2)/1 -> Product1/1

== system EiH_VFC_Renew_R2021b/Image Jacobian fco/eeo WS ==
  eeo : Inport
  Clock : Clock
  Demux4 : Demux  Outputs=6
      settings: DisplayOption=none
  Mux2 : Mux  Inputs=7
  To Workspace1 : ToWorkspace  VariableName=eeo  SaveFormat=Structure  SampleTime=-1
  wires:
  Demux4/6 -> Mux2/7
  Demux4/5 -> Mux2/6
  Demux4/4 -> Mux2/5
  Demux4/3 -> Mux2/4
  Demux4/2 -> Mux2/3
  Demux4/1 -> Mux2/2
  Clock/1 -> Mux2/1
  Mux2/1 -> To Workspace1/1
  eeo/1 -> Demux4/1

== system EiH_VFC_Renew_R2021b/Image Jacobian fco/maka ee ==
  J_daggar : Inport
  f : Inport  Port=2
  f_bar : Inport  Port=3
  Product4 : Product  Multiplication=Matrix(*)  InputSameDT=on  SaturateOnIntegerOverflow=on  OutDataTypeStr=Inherit: Same as first input
  Sum : Sum  Inputs=|+-  InputSameDT=on  SaturateOnIntegerOverflow=on  OutDataTypeStr=Inherit: Same as first input
  ee : Outport  VectorParamsAs1DForOutWhenUnconnected=off
  wires:
  f_bar/1 -> Sum/2
  f/1 -> Sum/1
  Product4/1 -> ee/1
  J_daggar/1 -> Product4/1
  Sum/1 -> Product4/2

== system EiH_VFC_Renew_R2021b/Image Jacobian fco/pseudo inverse ==
  J : Inport
  J^T : Math  Operator=transpose  SignedPower=on  SaturateOnIntegerOverflow=on
  J^T1 : Math  Operator=transpose  SignedPower=on  SaturateOnIntegerOverflow=on
  Product1 : Product  Inputs=/  Multiplication=Matrix(*)  InputSameDT=on  SaturateOnIntegerOverflow=on  OutDataTypeStr=Inherit: Same as first input
  Product2 : Product  Multiplication=Matrix(*)  InputSameDT=on  SaturateOnIntegerOverflow=on  OutDataTypeStr=Inherit: Same as first input
  Product4 : Product  Multiplication=Matrix(*)  InputSameDT=on  SaturateOnIntegerOverflow=on  OutDataTypeStr=Inherit: Same as first input
  J_daggar : Outport  VectorParamsAs1DForOutWhenUnconnected=off
  wires:
  Product2/1 -> J_daggar/1
  J^T1/1 -> Product2/2
  Product1/1 -> Product2/1
  Product4/1 -> Product1/1
  J^T/1 -> Product4/1
  J/1 -> J^T1/1, Product4/2, J^T/1

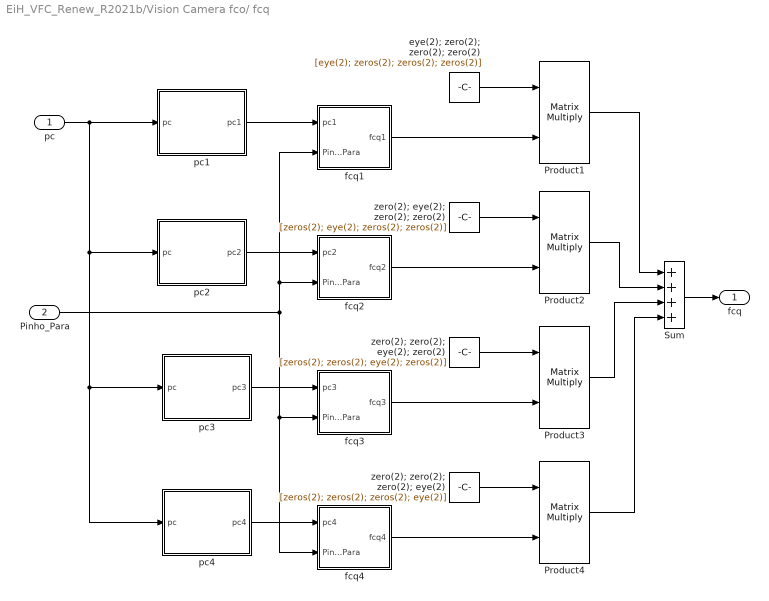
== system EiH_VFC_Renew_R2021b/Vision Camera fco/ fcq  ==
  pc : Inport
  Pinho_Para : Inport  Port=2
  Product{1..4} (4 alike) : Product  Multiplication=Matrix(*)  InputSameDT=on  SaturateOnIntegerOverflow=on  OutDataTypeStr=Inherit: Same as first input
  Sum : Sum  Inputs=++++  InputSameDT=on  SaturateOnIntegerOverflow=on  OutDataTypeStr=Inherit: Same as first input
  eye(2); zero(2); zero(2); zero(2) : Constant  Value=[eye(2); zeros(2); zeros(2); zeros(2)]  VectorParams1D=off
  fcq1 : Subsystem
  fcq2 : Subsystem
  fcq3 : Subsystem
  fcq4 : Subsystem
  pc1 : Subsystem
  pc2 : Subsystem
  pc3 : Subsystem
  pc4 : Subsystem
  zero(2); eye(2); zero(2); zero(2) : Constant  Value=[zeros(2); eye(2); zeros(2); zeros(2)]  VectorParams1D=off
  zero(2); zero(2); eye(2); zero(2) : Constant  Value=[zeros(2); zeros(2); eye(2); zeros(2)]  VectorParams1D=off
  zero(2); zero(2); zero(2); eye(2) : Constant  Value=[zeros(2); zeros(2); zeros(2); eye(2)]  VectorParams1D=off
  fcq : Outport  VectorParamsAs1DForOutWhenUnconnected=off
  wires:
  Pinho_Para/1 -> fcq4/2(Pinho_Para), fcq3/2(Pinho_Para), fcq2/2(Pinho_Para), fcq1/2(Pinho_Para)
  pc4/1(pc4) -> fcq4/1(pc4)
  pc3/1(pc3) -> fcq3/1(pc3)
  pc2/1(pc2) -> fcq2/1(pc2)
  Sum/1 -> fcq/1
  fcq4/1(fcq4) -> Product4/2
  fcq3/1(fcq3) -> Product3/2
  fcq2/1(fcq2) -> Product2/2
  fcq1/1(fcq1) -> Product1/2
  Product4/1 -> Sum/4
  Product2/1 -> Sum/2
  Product3/1 -> Sum/3
  Product1/1 -> Sum/1
  zero(2); zero(2); zero(2); eye(2)/1 -> Product4/1
  zero(2); zero(2); eye(2); zero(2)/1 -> Product3/1
  zero(2); eye(2); zero(2); zero(2)/1 -> Product2/1
  eye(2); zero(2); zero(2); zero(2)/1 -> Product1/1
  pc/1 -> pc4/1(pc), pc3/1(pc), pc2/1(pc), pc1/1(pc)
  pc1/1(pc1) -> fcq1/1(pc1)

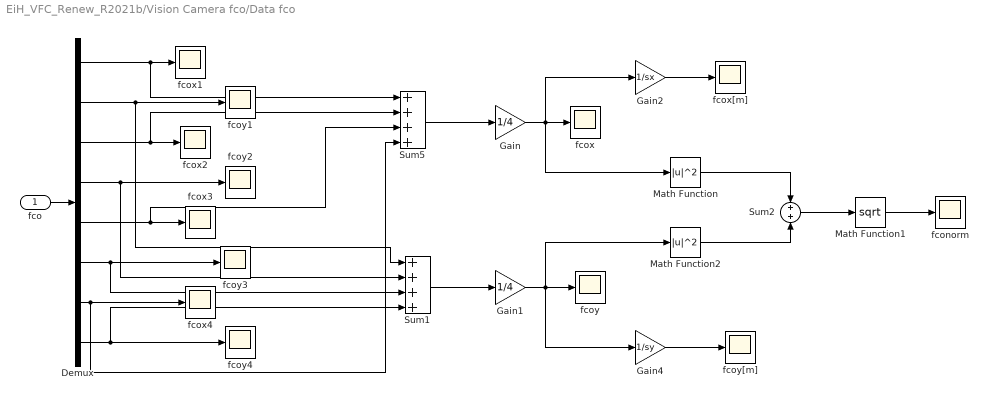
== system EiH_VFC_Renew_R2021b/Vision Camera fco/Data fco ==
  fco : Inport
  Demux : Demux  Outputs=8
      settings: DisplayOption=none
  Gain : Gain  Gain=1/4  SaturateOnIntegerOverflow=on  OutDataTypeStr=Inherit: Same as input  ParamDataTypeStr=Inherit: Same as input
  Gain1 : Gain  Gain=1/4  SaturateOnIntegerOverflow=on  OutDataTypeStr=Inherit: Same as input  ParamDataTypeStr=Inherit: Same as input
  Gain2 : Gain  Gain=1/sx  SaturateOnIntegerOverflow=on  OutDataTypeStr=Inherit: Same as input  ParamDataTypeStr=Inherit: Same as input
  Gain4 : Gain  Gain=1/sy  SaturateOnIntegerOverflow=on  OutDataTypeStr=Inherit: Same as input  ParamDataTypeStr=Inherit: Same as input
  Math Function : Math  Operator=magnitude^2  SignedPower=on  SaturateOnIntegerOverflow=on
  Math Function1 : Math  Operator=sqrt  SignedPower=on  SaturateOnIntegerOverflow=on
  Math Function2 : Math  Operator=magnitude^2  SignedPower=on  SaturateOnIntegerOverflow=on
  Sum1 : Sum  Inputs=++++  SaturateOnIntegerOverflow=on
  Sum2 : Sum  Inputs=+|+  SaturateOnIntegerOverflow=on
  Sum5 : Sum  Inputs=++++  SaturateOnIntegerOverflow=on
  fconorm : Scope
  fcox{,1..4} (5 alike) : Scope
  fcox[m] : Scope
  fcoy{,1..4} (5 alike) : Scope
  fcoy[m] : Scope
  wires:
  Gain4/1 -> fcoy[m]/1
  Gain2/1 -> fcox[m]/1
  Math Function1/1 -> fconorm/1
  Sum2/1 -> Math Function1/1
  Math Function2/1 -> Sum2/2
  Math Function/1 -> Sum2/1
  Gain1/1 -> Gain4/1, Math Function2/1, fcoy/1
  Sum1/1 -> Gain1/1
  Gain/1 -> Gain2/1, Math Function/1, fcox/1
  Sum5/1 -> Gain/1
  Demux/8 -> fcoy4/1, Sum1/4
  Demux/7 -> Sum5/4, fcox4/1
  Demux/6 -> Sum1/3, fcoy3/1
  Demux/5 -> Sum5/3, fcox3/1
  Demux/3 -> Sum5/2, fcox2/1
  fco/1 -> Demux/1
  Demux/2 -> Sum1/1, fcoy1/1
  Demux/1 -> Sum5/1, fcox1/1
  Demux/4 -> Sum1/2, fcoy2/1

== system EiH_VFC_Renew_R2021b/Vision Camera fco/Feature Point Model ==
  pcq : Inport
  Rcq : Inport  Port=2
  pq : Inport  Port=3
  Product{1..4} (4 alike) : Product  Multiplication=Matrix(*)  InputSameDT=on  SaturateOnIntegerOverflow=on  OutDataTypeStr=Inherit: Same as first input
  Sum : Sum  Inputs=++++  InputSameDT=on  SaturateOnIntegerOverflow=on  OutDataTypeStr=Inherit: Same as first input
  eye(3); zero(3); zero(3); zero(3) : Constant  Value=[eye(3); zeros(3); zeros(3); zeros(3)]  VectorParams1D=off
  pc1 : Subsystem
  pc2 : Subsystem
  pc3 : Subsystem
  pc4 : Subsystem
  zero(3); eye(3); zero(3); zero(3) : Constant  Value=[zeros(3); eye(3); zeros(3); zeros(3)]  VectorParams1D=off
  zero(3); zero(3); eye(3); zero(3) : Constant  Value=[zeros(3); zeros(3); eye(3); zeros(3)]  VectorParams1D=off
  zero(3); zero(3); zero(3); eye(3) : Constant  Value=[zeros(3); zeros(3); zeros(3); eye(3)]  VectorParams1D=off
  pc : Outport  VectorParamsAs1DForOutWhenUnconnected=off
  wires:
  Product4/1 -> Sum/4
  Product2/1 -> Sum/2
  Product3/1 -> Sum/3
  Product1/1 -> Sum/1
  Sum/1 -> pc/1
  pc4/1(pc4) -> Product4/2
  zero(3); zero(3); zero(3); eye(3)/1 -> Product4/1
  pc3/1(pc3) -> Product3/2
  zero(3); zero(3); eye(3); zero(3)/1 -> Product3/1
  pc2/1(pc2) -> Product2/2
  zero(3); eye(3); zero(3); zero(3)/1 -> Product2/1
  pc1/1(pc1) -> Product1/2
  eye(3); zero(3); zero(3); zero(3)/1 -> Product1/1
  pq/1 -> pc4/3(pq), pc3/3(pq), pc2/3(pq), pc1/3(pq)
  pcq/1 -> pc4/1(pcq), pc3/1(pcq), pc2/1(pcq), pc1/1(pcq)
  Rcq/1 -> pc4/2(Rcq), pc3/2(Rcq), pc2/2(Rcq), pc1/2(Rcq)

== system EiH_VFC_Renew_R2021b/Vision Camera fco/fco WS ==
  fco : Inport
  Clock : Clock
  Demux4 : Demux  Outputs=8
      settings: DisplayOption=none
  Mux2 : Mux  Inputs=9
  To Workspace1 : ToWorkspace  VariableName=fco  SaveFormat=Structure  SampleTime=-1
  wires:
  fco/1 -> Demux4/1
  Mux2/1 -> To Workspace1/1
  Clock/1 -> Mux2/1
  Demux4/1 -> Mux2/2
  Demux4/2 -> Mux2/3
  Demux4/3 -> Mux2/4
  Demux4/4 -> Mux2/5
  Demux4/5 -> Mux2/6
  Demux4/6 -> Mux2/7
  Demux4/7 -> Mux2/8
  Demux4/8 -> Mux2/9

== system EiH_VFC_Renew_R2021b/Vision Camera fco/make pzeta co ==
  "pco " : Inport
  Rco : Inport  Port=2
  Data pco1 : Subsystem
  Data zetaco : Subsystem
  "Rco -> zeta_co" : Subsystem
  pco WS : Subsystem
  zeta co WS : Subsystem
  wires:
  "pco "/1 -> pco WS/1(pco), Data pco1/1("pco ")
  Rco/1 -> "Rco -> zeta_co"/1(Rco)
  "Rco -> zeta_co"/1(zeta_co) -> zeta co WS/1(zetaco), Data zetaco/1(zetaco)

== system EiH_VFC_Renew_R2021b/Vwo Object/Data Vwo ==
  Vwo : Inport
  Demux4 : Demux  Outputs=6
      settings: DisplayOption=none
  omega_wox : Scope
  omega_woy : Scope
  omega_woz : Scope
  v_wox : Scope
  v_woy : Scope
  v_woz : Scope
  wires:
  Demux4/1 -> v_wox/1
  Demux4/2 -> v_woy/1
  Demux4/3 -> v_woz/1
  Demux4/4 -> omega_wox/1
  Demux4/5 -> omega_woy/1
  Demux4/6 -> omega_woz/1
  Vwo/1 -> Demux4/1

== system EiH_VFC_Renew_R2021b/Vwo Object/Data pwo ==
  pwo : Inport
  Demux4 : Demux  Outputs=3
      settings: DisplayOption=none
  pwo_x : Scope
  pwo_y : Scope
  pwo_z : Scope
  wires:
  Demux4/1 -> pwo_x/1
  Demux4/2 -> pwo_y/1
  Demux4/3 -> pwo_z/1
  pwo/1 -> Demux4/1

== system EiH_VFC_Renew_R2021b/Vwo Object/Data zetawo ==
  zeta wo : Inport
  Demux4 : Demux  Outputs=3
      settings: DisplayOption=none
  zetawo_x : Scope
  zetawo_y : Scope
  zetawo_z : Scope
  wires:
  Demux4/1 -> zetawo_x/1
  Demux4/2 -> zetawo_y/1
  Demux4/3 -> zetawo_z/1
  zeta wo/1 -> Demux4/1

== system EiH_VFC_Renew_R2021b/Vwo Object/Vwo WS ==
  Vwo : Inport
  Clock : Clock
  Demux4 : Demux  Outputs=6
      settings: DisplayOption=none
  Mux2 : Mux  Inputs=7
  To Workspace1 : ToWorkspace  VariableName=Vwo  SaveFormat=Structure  SampleTime=-1
  wires:
  Vwo/1 -> Demux4/1
  Mux2/1 -> To Workspace1/1
  Clock/1 -> Mux2/1
  Demux4/1 -> Mux2/2
  Demux4/2 -> Mux2/3
  Demux4/3 -> Mux2/4
  Demux4/4 -> Mux2/5
  Demux4/5 -> Mux2/6
  Demux4/6 -> Mux2/7

== system EiH_VFC_Renew_R2021b/Vwo Object/highspeed_exp_object_motion ==
  Clock : Clock
  Clock1 : Clock
  Clock2 : Clock
  Gain : Gain  Gain=pi/6  SaturateOnIntegerOverflow=on  OutDataTypeStr=Inherit: Same as input  ParamDataTypeStr=Inherit: Same as input
  MATLAB Fcn : MATLABFcn  MATLABFcn=highspeedmaketarget  OutputDimensions=6
  MATLAB Fcn1 : MATLABFcn  MATLABFcn=highspeedmakestraight  OutputDimensions=6
  Sum4 : Sum  Inputs=|+-  InputSameDT=on  SaturateOnIntegerOverflow=on  OutDataTypeStr=Inherit: Same as first input
  Switch : Switch  Threshold=2  SaturateOnIntegerOverflow=on
  Switch1 : Switch  Threshold=4.8  SaturateOnIntegerOverflow=on
  Terminator1 : Terminator
  Terminator2 : Terminator
  Terminator7 : Terminator
  arbitrary : Constant  Value=pzeta_wo_init  VectorParams1D=off
  t=14 : Constant  Value=[0.39856406460551;0;-1; 0;0;-0.50874321553273]  VectorParams1D=off
  t=2 : Constant  Value=[0.4678;0;-1;0;0;-0.2913]  VectorParams1D=off
  time : Constant  Value=2  VectorParams1D=off
  zero1 : Constant  Value=4.8  VectorParams1D=off
  pwo & xiwo : Outport  VectorParamsAs1DForOutWhenUnconnected=off
  wires:
  arbitrary/1 -> pwo & xiwo/1
  t=14/1 -> Terminator1/1
  Switch/1 -> Terminator7/1
  Clock1/1 -> Switch1/3, Switch1/2
  Switch1/1 -> Sum4/1
  zero1/1 -> Switch1/1
  Sum4/1 -> Gain/1
  time/1 -> Sum4/2
  MATLAB Fcn/1 -> Switch/1
  Gain/1 -> MATLAB Fcn/1
  Clock/1 -> Switch/2
  t=2/1 -> Terminator2/1
  Clock2/1 -> MATLAB Fcn1/1
  MATLAB Fcn1/1 -> Switch/3

== system EiH_VFC_Renew_R2021b/Vwo Object/pwo WS ==
  pwo : Inport
  Clock : Clock
  Demux4 : Demux  Outputs=3
      settings: DisplayOption=none
  Mux2 : Mux
  To Workspace1 : ToWorkspace  VariableName=pwo  SaveFormat=Structure  SampleTime=-1
  wires:
  Demux4/3 -> Mux2/4
  Demux4/2 -> Mux2/3
  Demux4/1 -> Mux2/2
  Clock/1 -> Mux2/1
  Mux2/1 -> To Workspace1/1
  pwo/1 -> Demux4/1

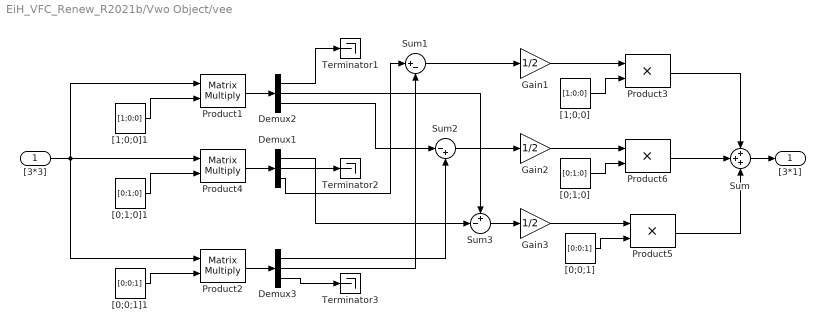
== system EiH_VFC_Renew_R2021b/Vwo Object/vee ==
  "[3*3]" : Inport
  Demux1 : Demux  Outputs=3
      settings: DisplayOption=none
  Demux2 : Demux  Outputs=3
      settings: DisplayOption=none
  Demux3 : Demux  Outputs=3
      settings: DisplayOption=none
  Gain1 : Gain  Gain=1/2  SaturateOnIntegerOverflow=on  OutDataTypeStr=Inherit: Same as input  ParamDataTypeStr=Inherit: Same as input
  Gain2 : Gain  Gain=1/2  SaturateOnIntegerOverflow=on  OutDataTypeStr=Inherit: Same as input  ParamDataTypeStr=Inherit: Same as input
  Gain3 : Gain  Gain=1/2  SaturateOnIntegerOverflow=on  OutDataTypeStr=Inherit: Same as input  ParamDataTypeStr=Inherit: Same as input
  Product1 : Product  Multiplication=Matrix(*)  InputSameDT=on  SaturateOnIntegerOverflow=on  OutDataTypeStr=Inherit: Same as first input
  Product2 : Product  Multiplication=Matrix(*)  InputSameDT=on  SaturateOnIntegerOverflow=on  OutDataTypeStr=Inherit: Same as first input
  Product3 : Product  InputSameDT=on  SaturateOnIntegerOverflow=on  OutDataTypeStr=Inherit: Same as first input
  Product4 : Product  Multiplication=Matrix(*)  InputSameDT=on  SaturateOnIntegerOverflow=on  OutDataTypeStr=Inherit: Same as first input
  Product5 : Product  InputSameDT=on  SaturateOnIntegerOverflow=on  OutDataTypeStr=Inherit: Same as first input
  Product6 : Product  InputSameDT=on  SaturateOnIntegerOverflow=on  OutDataTypeStr=Inherit: Same as first input
  Sum : Sum  Inputs=+++  InputSameDT=on  SaturateOnIntegerOverflow=on  OutDataTypeStr=Inherit: Same as first input
  Sum1 : Sum  Inputs=|+-  InputSameDT=on  SaturateOnIntegerOverflow=on  OutDataTypeStr=Inherit: Same as first input
  Sum2 : Sum  Inputs=|-+  InputSameDT=on  SaturateOnIntegerOverflow=on  OutDataTypeStr=Inherit: Same as first input
  Sum3 : Sum  Inputs=+-|  InputSameDT=on  SaturateOnIntegerOverflow=on  OutDataTypeStr=Inherit: Same as first input
  Terminator1 : Terminator
  Terminator2 : Terminator
  Terminator3 : Terminator
  "[0;0;1]" : Constant  Value=[0;0;1]  VectorParams1D=off
  "[0;0;1]1" : Constant  Value=[0;0;1]  VectorParams1D=off
  "[0;1;0]" : Constant  Value=[0;1;0]  VectorParams1D=off
  "[0;1;0]1" : Constant  Value=[0;1;0]  VectorParams1D=off
  "[1;0;0]" : Constant  Value=[1;0;0]  VectorParams1D=off
  "[1;0;0]1" : Constant  Value=[1;0;0]  VectorParams1D=off
  "[3*1]" : Outport  VectorParamsAs1DForOutWhenUnconnected=off
  wires:
  "[3*3]"/1 -> Product2/1, Product1/1, Product4/1
  "[0;1;0]1"/1 -> Product4/2
  Product4/1 -> Demux1/1
  Demux1/2 -> Terminator2/1
  Demux1/3 -> Sum1/1
  "[1;0;0]1"/1 -> Product1/2
  Product1/1 -> Demux2/1
  Demux2/1 -> Terminator1/1
  "[0;0;1]1"/1 -> Product2/2
  Product2/1 -> Demux3/1
  Demux3/3 -> Terminator3/1
  Demux3/1 -> Sum2/2
  "[1;0;0]"/1 -> Product3/2
  "[0;1;0]"/1 -> Product6/2
  "[0;0;1]"/1 -> Product5/2
  Product6/1 -> Sum/2
  Product5/1 -> Sum/3
  Product3/1 -> Sum/1
  Sum/1 -> "[3*1]"/1
  Sum1/1 -> Gain1/1
  Gain1/1 -> Product3/1
  Demux3/2 -> Sum1/2
  Gain2/1 -> Product6/1
  Gain3/1 -> Product5/1
  Demux2/3 -> Sum2/1
  Sum2/1 -> Gain2/1
  Sum3/1 -> Gain3/1
  Demux2/2 -> Sum3/1
  Demux1/1 -> Sum3/2

== system EiH_VFC_Renew_R2021b/Vwo Object/zetawo WS ==
  zetawo : Inport
  Clock : Clock
  Demux4 : Demux  Outputs=3
      settings: DisplayOption=none
  Mux2 : Mux
  To Workspace1 : ToWorkspace  VariableName=zetawo  SaveFormat=Structure  SampleTime=-1
  wires:
  zetawo/1 -> Demux4/1
  Clock/1 -> Mux2/1
  Mux2/1 -> To Workspace1/1
  Demux4/3 -> Mux2/4
  Demux4/2 -> Mux2/3
  Demux4/1 -> Mux2/2

== system EiH_VFC_Renew_R2021b/make Ad(ge)/wedge ==
  "[3x1]" : Inport
  Product1 : Product  InputSameDT=on  SaturateOnIntegerOverflow=on  OutDataTypeStr=Inherit: Same as first input
  Product2 : Product  InputSameDT=on  SaturateOnIntegerOverflow=on  OutDataTypeStr=Inherit: Same as first input
  Product3 : Product  InputSameDT=on  SaturateOnIntegerOverflow=on  OutDataTypeStr=Inherit: Same as first input
  Sum : Sum  Inputs=+++  InputSameDT=on  SaturateOnIntegerOverflow=on  OutDataTypeStr=Inherit: Same as first input
  Xaxis : Constant  Value=[0 0 0;0 0 -1;0 1 0]  VectorParams1D=off
  Yaxis : Constant  Value=[0 0 1;0 0 0;-1 0 0]  VectorParams1D=off
  Zaxis : Constant  Value=[0 -1 0;1 0 0;0 0 0]  VectorParams1D=off
  x : Gain  Gain=[1 0 0]  Multiplication=Matrix(K*u)  SaturateOnIntegerOverflow=on  OutDataTypeStr=Inherit: Same as input  ParamDataTypeStr=Inherit: Same as input
  y : Gain  Gain=[0 1 0]  Multiplication=Matrix(K*u)  SaturateOnIntegerOverflow=on  OutDataTypeStr=Inherit: Same as input  ParamDataTypeStr=Inherit: Same as input
  z : Gain  Gain=[0 0 1]  Multiplication=Matrix(K*u)  SaturateOnIntegerOverflow=on  OutDataTypeStr=Inherit: Same as input  ParamDataTypeStr=Inherit: Same as input
  "[3x3]" : Outport  VectorParamsAs1DForOutWhenUnconnected=off
  wires:
  Sum/1 -> "[3x3]"/1
  Product1/1 -> Sum/3
  Product2/1 -> Sum/1
  Product3/1 -> Sum/2
  "[3x1]"/1 -> z/1, x/1, y/1
  y/1 -> Product3/1
  Yaxis/1 -> Product3/2
  x/1 -> Product2/1
  Xaxis/1 -> Product2/2
  z/1 -> Product1/1
  Zaxis/1 -> Product1/2
